simulink model "solarfuzzympptbldcmotorbattery"  (R2016a)
settings: Solver=ode45  StartTime=0.0  StopTime=1  RelTol=1e-3
undefined symbols (not defined in the file): Ion, Lithium
libraries: powerlib x32, simulink x13, electricdrivelib x1, fuzblock x1
settings Model: Creator=sudheer  LastModifiedBy=sudheer
settings SolverCC: ZeroCrossAlgorithm=Adaptive

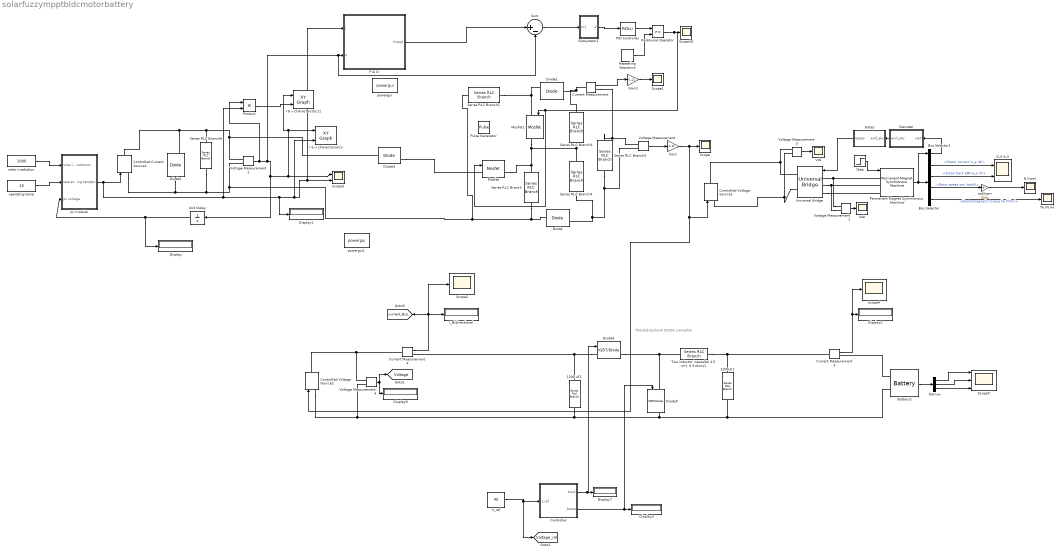
== system solarfuzzympptbldcmotorbattery ==
  note: The bidirectional DC/DC converter
  1200 uF1 : powerlib/Elements/Series RLC Branch  LConnTagsString=__new0  RConnTagsString=__new0  BranchType=RC  Resistance=0.001  Inductance=3e-3  SetiL0=off  InitialCurrent=0  Capacitance=1200e-6  Setx0=off  InitialVoltage=0  Measurements=None
  1200uF1 : powerlib/Elements/Series RLC Branch  LConnTagsString=__new0  RConnTagsString=__new0  BranchType=C  Resistance=1  Inductance=3e-3  SetiL0=off  InitialCurrent=0  Capacitance=1200e-6  Setx0=off  InitialVoltage=0  Measurements=None
  Battery2 : electricdrivelib/Extra Sources/Battery  BatType=Lithium-Ion  ShowTempParam=off  ThermalPreset=no  NomV=200  NomQ=100  SOC=80  Batt_Tr=0.1  PresetModel=on  MaxQ=100  MinV=150  FullV=232.7974  Dis_rate=43.4783  R=0.02  Normal_OP=90.4348  expZone="[216.0772      4.913043]"  current=[1.5 3]  Units=Ampere-hour  Tci=20  NomT=20  T2=-30  MaxQ2=4.8  FullV2=7.1  Normal_OP2=5.72  expZone2="[6.58  1]"  Rca=0.6  ti=1000  Dp=0
  Bus Selector : BusSelector  OutputSignals=Stator current is_a (A),Stator back EMF e_a (V),Rotor speed wm (rad/s),Electromagnetic torque Te (N*m)
  Bus Selector1 : BusSelector  OutputSignals=Hall effect signal h_a,Hall effect signal h_b,Hall effect signal h_c  OutputAsBus=on
  Controlled Current Source1 : powerlib/Electrical Sources/Controlled Current Source  Initialize=on  Source_Type=AC  Amplitude=0  Phase=0  Frequency=0  Measurements=None
  Controlled Voltage Source1 : powerlib/Electrical Sources/Controlled Voltage Source  Initialize=on  Source_Type=AC  Amplitude=500  Phase=0  Frequency=0  Measurements=None
  Controlled Voltage Source2 : powerlib/Electrical Sources/Controlled Voltage Source  Initialize=on  Source_Type=AC  Amplitude=500  Phase=0  Frequency=0  Measurements=None
  Controller : Subsystem
  Current Measurement : powerlib/Measurements/Current Measurement  PhasorSimulation=off  OutputType=Complex  PSBequivalent=0
  Current Measurement3 : powerlib/Measurements/Current Measurement  PhasorSimulation=off  OutputType=Complex  PSBequivalent=0
  Current Measurement4 : powerlib/Measurements/Current Measurement  PhasorSimulation=off  OutputType=Complex  PSBequivalent=0
  Decoder : Subsystem
  Demux : Demux  Outputs=3
  Diode{,1..3} (4 alike) : powerlib/Power Electronics/Diode  Ron=0.001  Lon=0  Vf=0.8  IC=0  UseSnubber=off  Rs=500  Cs=250e-9  Measurements=on
  Diode4 : powerlib/Power Electronics/IGBT//Diode  Ron=1e-3  Rs=1e5  Cs=inf  Measurements=on
  Diode5 : powerlib/Power Electronics/IGBT//Diode  Ron=1e-3  Rs=1e5  Cs=inf  Measurements=on
  Display{,1..3,7,9} (6 alike) : Display
  Gain : Gain  Gain=-1.11
  Gain1 : Gain  Gain=-1.11
  Gates : Subsystem
  I & v characteristics : simulink/Sinks/XY Graph  xmin=0  xmax=100  ymin=0  ymax=15  st=-1
  I & v characteristics1 : simulink/Sinks/XY Graph  xmin=0  xmax=100  ymin=0  ymax=1000  st=-1
  I_Bidirectional : Display
  Mosfet : powerlib/Power Electronics/Mosfet  Ron=0.1  Lon=0  Rd=0.01  Vfd=0  IC=0  Rs=1e5  Cs=inf  Measurements=on
  Mosfet1 : powerlib/Power Electronics/Mosfet  Ron=0.1  Lon=0  Rd=0.01  Vfd=0  IC=0  Rs=1e5  Cs=inf  Measurements=on
  N (rpm) : Scope
  P & O : Subsystem
  PID Controller : simulink/Continuous/PID Controller  Controller=PID  TimeDomain=Continuous-time  SampleTime=-1  IntegratorMethod=Forward Euler  FilterMethod=Forward Euler  Form=Parallel  UseFilter=on  ControllerParametersSource=internal  P=65  I=1300  D=1.1  N=1000  InitialConditionSource=internal  InitialConditionForIntegrator=0  InitialConditionForFilter=0  ExternalReset=none  LimitOutput=on  UpperSaturationLimit=0.9  LowerSaturationLimit=0.1  LinearizeAsGain=on  AntiWindupMode=none  Kb=1  TrackingMode=off  Kt=1  PParamMin=[]  PParamMax=[]  IParamMin=[]  IParamMax=[]  DParamMin=[]  DParamMax=[]  NParamMin=[]  NParamMax=[]  KbParamMin=[]  KbParamMax=[]  KtParamMin=[]  KtParamMax=[]  POutMin=[]  POutMax=[]  IOutMin=[]  IOutMax=[]  DOutMin=[]  DOutMax=[]  NOutMin=[]  NOutMax=[]  KbOutMin=[]  KbOutMax=[]  KtOutMin=[]  KtOutMax=[]  IntegratorOutMin=[]  IntegratorOutMax=[]  FilterOutMin=[]  FilterOutMax=[]  SumOutMin=[]  SumOutMax=[]  SumI1OutMin=[]  SumI1OutMax=[]  SumI2OutMin=[]  SumI2OutMax=[]  SumI3OutMin=[]  SumI3OutMax=[]  SumDOutMin=[]  SumDOutMax=[]  SaturationOutMin=[]  SaturationOutMax=[]  IntegratorContinuousStateAttributes=''  IntegratorStateMustResolveToSignalObject=off  IntegratorRTWStateStorageClass=Auto  FilterContinuousStateAttributes=''  FilterStateMustResolveToSignalObject=off  FilterRTWStateStorageClass=Auto  DifferentiatorICPrevScaledInput=0  DifferentiatorOutMin=[]  DifferentiatorOutMax=[]
  Permanent Magnet Synchronous Machine : powerlib/Machines/Permanent Magnet Synchronous Machine  NbPhases=3  FluxDistribution=Trapezoidal  RotorType=Round  MechanicalLoad=Torque Tm  PresetModel=No  ShowDetailedParameters=on  MeasurementBus=off  Resistance=2.8750  Inductance=8.5e-3  dqInductances=[8.5e-3, 8.5e-3]  La=0.000835  MachineConstant=Flux linkage established by magnets (V.s)  Flux=0.175  VoltageCst=146.6077  TorqueCst=1.4  Flat=120  Mechanical=[ 0.8e-3, 1e-3 4]  PolePairs=4  InitialConditions=[0,0, 0,0]  InitialConditions5ph=[0 0 0 0 0 0]  TsPowergui=0  TsBlock=-1  RefAngle=90 degrees behind phase A axis (modified Park)
  Product : Product
  Pulse Generator : DiscretePulseGenerator  PulseType=Time based  Period=1/24000  PulseWidth=70
  Relational Operator : RelationalOperator  OutDataTypeStr=boolean
  Repeating Sequence : simulink/Sources/Repeating Sequence  rep_seq_t=[0 1 2 3 4 ]*(1/3e3)  rep_seq_y=[0 1 0 -1 0]
  Scope{,1..2,4,16} (5 alike) : Scope
  Scope3 : Scope  NumInputPorts=2
  Scope5 : Scope  NumInputPorts=3
  Series RLC Branch : powerlib/Elements/Series RLC Branch  LConnTagsString=__new0  RConnTagsString=__new0  BranchType=L  Resistance=1  Inductance=1e-3  SetiL0=off  InitialCurrent=0  Capacitance=1e-6  Setx0=off  InitialVoltage=0  Measurements=None
  Series RLC Branch1 : powerlib/Elements/Series RLC Branch  LConnTagsString=__new0  RConnTagsString=__new0  BranchType=C  Resistance=1  Inductance=1e-3  SetiL0=off  InitialCurrent=0  Capacitance=500e-6  Setx0=off  InitialVoltage=0  Measurements=None
  Series RLC Branch2 : powerlib/Elements/Series RLC Branch  LConnTagsString=__new0  RConnTagsString=__new0  BranchType=R  Resistance=100  Inductance=1e-3  SetiL0=off  InitialCurrent=0  Capacitance=1e-6  Setx0=off  InitialVoltage=0  Measurements=None
  Series RLC Branch3 : powerlib/Elements/Series RLC Branch  LConnTagsString=__new0  RConnTagsString=__new0  BranchType=C  Resistance=1  Inductance=1e-3  SetiL0=off  InitialCurrent=0  Capacitance=300e-6  Setx0=off  InitialVoltage=0  Measurements=None
  Series RLC Branch4 : powerlib/Elements/Series RLC Branch  LConnTagsString=__new0  RConnTagsString=__new0  BranchType=C  Resistance=1  Inductance=1e-3  SetiL0=off  InitialCurrent=0  Capacitance=300e-6  Setx0=off  InitialVoltage=0  Measurements=None
  Series RLC Branch6 : powerlib/Elements/Series RLC Branch  LConnTagsString=__new0  RConnTagsString=__new0  BranchType=C  Resistance=1  Inductance=1e-3  SetiL0=off  InitialCurrent=0  Capacitance=1000e-6  Setx0=on  InitialVoltage=0  Measurements=None
  Step : Step  Time=.1  After=3  SampleTime=0
  Subsystem1 : Subsystem
  Sum : Sum  Inputs=|+-
  Te (N.m) : Scope
  "Two inductor inparallel 4.5 mH, 0.3 ohms1" : powerlib/Elements/Series RLC Branch  LConnTagsString=__new0  RConnTagsString=__new0  BranchType=RL  Resistance=.25  Inductance=4.5e-3  SetiL0=off  InitialCurrent=0  Capacitance=1e-6  Setx0=off  InitialVoltage=0  Measurements=None
  Unit Delay : UnitDelay  SampleTime=-1
  Universal Bridge : powerlib/Power Electronics/Universal Bridge  Arms=3  SnubberResistance=5000  SnubberCapacitance=1e-6  Device=MOSFET / Diodes  Ron=1e-3  Lon=0  ForwardVoltages="[  0  0  ]"  ForwardVoltage=0  GTOparameters=[ 10e-6 , 20e-6 ]  IGBTparameters=[ 1e-6 , 2e-6 ]  Measurements=None  Measurements_2=None  converterType=Rectifier
  V_ref : Constant  Value=45
  Vab : Scope
  Vdc : Scope
  Voltage Measurement{,1..4} (5 alike) : powerlib/Measurements/Voltage Measurement  PhasorSimulation=off  OutputType=Complex  PSBequivalent=0
  is_a e_a : Scope  NumInputPorts=2
  operating temp : Constant  Value=25
  powergui : powerlib/powergui  Priority=1  SimulationMode=Discrete  SolverType=Tustin/Backward Euler (TBE)  SampleTime=50e-6  frequency=60  SPID=off  DisableSnubberDevices=off  DisableRonSwitches=off  DisableVfSwitches=off  SwTol=0  DisplayEquations=off  Interpol=off  ExternalGateDelay=off  methode=off  Ts=10  FunctionMessages=off  echomessages=off  HookPort=off  EnableUseOfTLC=off  x0status=blocks  frequencyindice=0  Pbase=100e6  ErrMax=1e-4  Iterations=50  UnitsV=kV  UnitsW=MW  buscounter=0  RestoreLinks=warning  ResistiveCurrentMeasurement=off  Frange=[0:2:500]  Ylog=off  Xlog=on  ShowGrid=off  save=off  variable=ZData  structure=0  ZoomFFT=off  StartTime=0.0  cycles=1  DisplayStyle=1  fundamental=60  FreqAxis=off  MaxFrequency=1000  frequencyindicesteady=1  RmsSteady=1  display=off
  powergui1 : powerlib/powergui  Priority=1  SimulationMode=Discrete  SolverType=Backward Euler  SampleTime=1e-5  frequency=60  SPID=off  DisableSnubberDevices=off  DisableRonSwitches=off  DisableVfSwitches=off  SwTol=0  DisplayEquations=off  Interpol=off  ExternalGateDelay=off  methode=off  Ts=0  FunctionMessages=off  echomessages=off  HookPort=off  EnableUseOfTLC=off  x0status=blocks  frequencyindice=0  Pbase=100e6  ErrMax=1e-4  Iterations=50  UnitsV=kV  UnitsW=MW  buscounter=0  RestoreLinks=warning  ResistiveCurrentMeasurement=off  Frange=[0:2:500]  Ylog=off  Xlog=on  ShowGrid=off  save=off  variable=ZData  structure=0  ZoomFFT=off  StartTime=0.0  cycles=1  DisplayStyle=1  fundamental=60  FreqAxis=off  MaxFrequency=1000  frequencyindicesteady=1  RmsSteady=1  display=off
  pv module : Subsystem  mask{Voc=60, Isc=9.4, Ns=100, Np=1, Rsh=1000, Rs=0.0001}
      mask prompts: Voc "open circuit voltage"; Isc "shortcircuit current"; Ns "modules in series"; Np "modules in parallel"; Rsh "shunt resistance"; Rs "series resistance"
  rad2rpm : Gain  Gain=30/pi
  solar irradiation : Constant  Value=1000
  tag scope: Voltage=global, Voltage_ref=global, current_Bus=global
  wires:
  Voltage Measurement/1 -> Gain/1
  Current Measurement/1 -> Gain1/1
  Gain/1 -> Controlled Voltage Source2/1, Controlled Voltage Source1/1, Scope/1
  solar irradiation/1 -> pv module/1(solar irradiation)
  operating temp/1 -> pv module/2(operating temp)
  Voltage Measurement1/1 -> Product/1, Sum/2, P & O/2(V), I & v characteristics/1, I & v characteristics1/1, Scope3/1, Unit Delay/1
  Unit Delay/1 -> Display/1, pv module/3(pv voltage)
  pv module/1(Ipv) -> Display1/1, I & v characteristics/2, Scope3/2, P & O/1(I), Product/2, Controlled Current Source1/1
  P & O/1(Vmpp1) -> Sum/1
  Relational Operator/1 -> Mosfet/1, Mosfet1/1, Scope16/1
  Sum/1 -> Subsystem1/1(In1)
  Repeating Sequence/1 -> Relational Operator/2
  PID Controller/1 -> Relational Operator/1
  Subsystem1/1(Out1) -> PID Controller/1
  Step/1 -> Permanent Magnet Synchronous Machine/1
  Gates/1(Gates) -> Universal Bridge/1
  Decoder/1(emf_abc) -> Gates/1("emf_abc ")
  rad2rpm/1 -> N (rpm)/1
  Voltage Measurement2/1 -> Vab/1
  Voltage Measurement3/1 -> Vdc/1
  Bus Selector/1 -> is_a e_a/1  "<Stator current is_a (A)>"
  Permanent Magnet Synchronous Machine/1 -> Bus Selector/1, Bus Selector1/1
  Bus Selector1/1 -> Decoder/1("Hall ")
  Bus Selector/2 -> is_a e_a/2  "<Stator back EMF e_a (V)>"
  Bus Selector/3 -> rad2rpm/1  "<Rotor speed wm (rad/s)>"
  Bus Selector/4 -> Te (N.m)/1  "<Electromagnetic torque Te (N*m)>"
  Current Measurement3/1 -> Display2/1, Scope4/1
  Controller/2(boost) -> Diode5/1, Display3/1
  Controller/1(buck) -> Diode4/1, Display7/1
  Current Measurement4/1 -> [current_Bus], Scope2/1, I_Bidirectional/1
  Voltage Measurement4/1 -> Display9/1, [Voltage]
  V_ref/1 -> [Voltage_ref], Controller/1(I_ref)
  Battery2/1 -> Demux/1
  Demux/1 -> Scope5/1
  Demux/2 -> Scope5/2
  Demux/3 -> Scope5/3
  Gain1/1 -> Scope1/1
  Product/1 -> I & v characteristics1/2
  connections:
  Voltage Measurement4/LConn1 -- Current Measurement4/LConn1 -- Controlled Voltage Source2/RConn1
  Series RLC Branch1/RConn1 -- Diode1/RConn1 -- Mosfet1/LConn1
  Universal Bridge/RConn1 -- Controlled Voltage Source1/RConn1 -- Voltage Measurement3/LConn1
  Series RLC Branch2/RConn1 -- Voltage Measurement/LConn2 -- Series RLC Branch4/LConn1 -- Diode/RConn1
  Current Measurement/LConn1 -- Series RLC Branch3/RConn1 -- Diode1/LConn1
  Diode5/RConn1 -- Controlled Voltage Source2/LConn1 -- Voltage Measurement4/LConn2 -- 1200 uF1/RConn1 -- Battery2/LConn2 -- 1200uF1/RConn1
  Controlled Current Source1/RConn1 -- Diode2/RConn1 -- Diode3/LConn1 -- Voltage Measurement1/LConn1 -- Series RLC Branch6/LConn1
  Diode3/RConn1 -- Mosfet/LConn1
  Voltage Measurement2/LConn1 -- Permanent Magnet Synchronous Machine/LConn1 -- Universal Bridge/LConn1
  Voltage Measurement2/LConn2 -- Permanent Magnet Synchronous Machine/LConn2 -- Universal Bridge/LConn2
  Universal Bridge/LConn3 -- Permanent Magnet Synchronous Machine/LConn3
  Series RLC Branch2/LConn1 -- Current Measurement/RConn1 -- Voltage Measurement/LConn1
  Universal Bridge/RConn2 -- Controlled Voltage Source1/LConn1 -- Voltage Measurement3/LConn2
  "Two inductor inparallel 4.5 mH, 0.3 ohms1"/LConn1 -- Diode5/LConn1 -- Diode4/RConn1
  1200uF1/LConn1 -- Current Measurement3/LConn1 -- "Two inductor inparallel 4.5 mH, 0.3 ohms1"/RConn1
  Diode4/LConn1 -- 1200 uF1/LConn1 -- Current Measurement4/RConn1
  Battery2/LConn1 -- Current Measurement3/RConn1
  Mosfet/RConn1 -- Mosfet1/RConn1 -- Series RLC Branch3/LConn1 -- Series RLC Branch4/RConn1 -- Series RLC Branch/LConn1
  Voltage Measurement1/LConn2 -- Series RLC Branch/RConn1 -- Diode/LConn1 -- Series RLC Branch1/LConn1 -- Series RLC Branch6/RConn1 -- Diode2/LConn1 -- Controlled Current Source1/LConn1

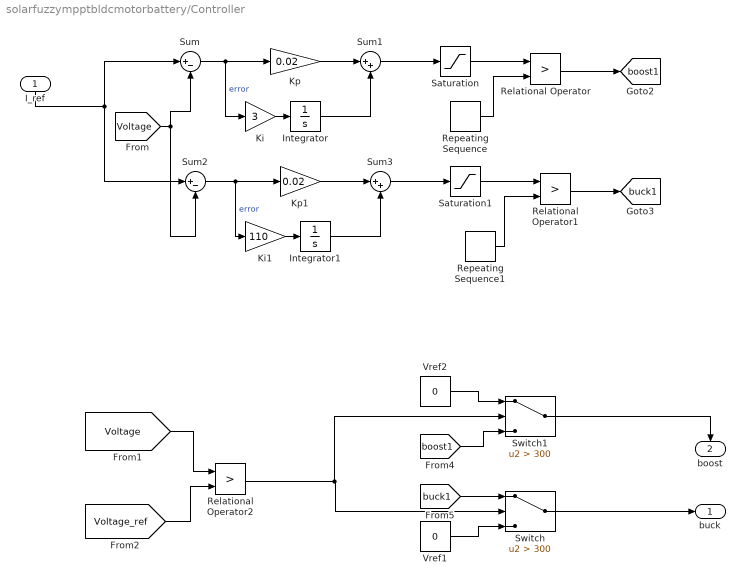
== system solarfuzzympptbldcmotorbattery/Controller ==
  I_ref : Inport
  Integrator : Integrator  LimitOutput=on  UpperSaturationLimit=0.9  LowerSaturationLimit=0
  Integrator1 : Integrator  LimitOutput=on  UpperSaturationLimit=0.9  LowerSaturationLimit=0
  Ki : Gain  Gain=3
  Ki1 : Gain  Gain=110
  Kp : Gain  Gain=0.02
  Kp1 : Gain  Gain=0.02
  Relational Operator : RelationalOperator  Operator=>  OutDataTypeStr=boolean
  Relational Operator1 : RelationalOperator  Operator=>  OutDataTypeStr=boolean
  Relational Operator2 : RelationalOperator  Operator=>  OutDataTypeStr=boolean
  Repeating Sequence : simulink/Sources/Repeating Sequence  rep_seq_t=[0 1/5000]  rep_seq_y=[0 1]
  Repeating Sequence1 : simulink/Sources/Repeating Sequence  rep_seq_t=[0 1/5000]  rep_seq_y=[0 1]
  Saturation : Saturate  UpperLimit=0.9  LowerLimit=0
  Saturation1 : Saturate  UpperLimit=0.9  LowerLimit=0
  Sum : Sum  Inputs=|+-
  Sum1 : Sum  Inputs=|++
  Sum2 : Sum  Inputs=|+-
  Sum3 : Sum  Inputs=|++
  Switch : Switch  Criteria=u2 > Threshold  Threshold=300
  Switch1 : Switch  Criteria=u2 > Threshold  Threshold=300
  Vref1 : Constant  Value=0
  Vref2 : Constant  Value=0
  buck : Outport
  boost : Outport  Port=2
  tag scope: boost1=global, buck1=global
  wires:
  Switch/1 -> buck/1
  [boost1] -> Switch1/3
  Switch1/1 -> boost/1
  Ki1/1 -> Integrator1/1
  Saturation1/1 -> Relational Operator1/1
  Saturation/1 -> Relational Operator/1
  Sum2/1 -> Kp1/1, Ki1/1  "error"
  Relational Operator1/1 -> [buck1]
  Kp1/1 -> Sum3/1
  [Voltage] -> Sum2/2, Sum/2
  Repeating Sequence1/1 -> Relational Operator1/2
  Repeating Sequence/1 -> Relational Operator/2
  Integrator1/1 -> Sum3/2
  Sum3/1 -> Saturation1/1
  Ki/1 -> Integrator/1
  Sum1/1 -> Saturation/1
  I_ref/1 -> Sum/1, Sum2/1
  Relational Operator/1 -> [boost1]
  Sum/1 -> Ki/1, Kp/1  "error"
  Kp/1 -> Sum1/1
  Integrator/1 -> Sum1/2
  Vref2/1 -> Switch1/1
  Vref1/1 -> Switch/3
  [buck1] -> Switch/1
  [Voltage] -> Relational Operator2/1
  [Voltage_ref] -> Relational Operator2/2
  Relational Operator2/1 -> Switch1/2, Switch/2

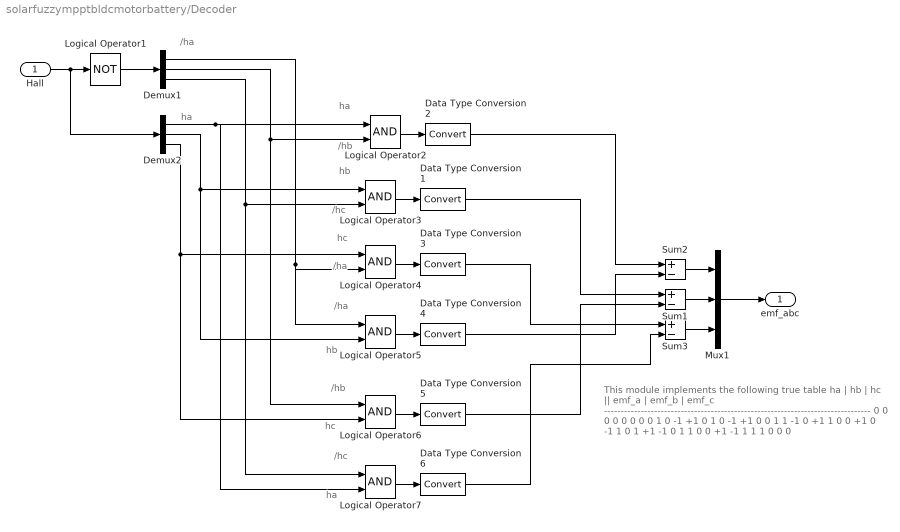
== system solarfuzzympptbldcmotorbattery/Decoder ==
  note: /ha
  note: ha
  note: ha
  note: /hb
  note: hb
  note: /hc
  note: hc
  note: /ha
  note: /ha
  note: hb
  note: /hb
  note: hc
  note: /hc
  note: ha
  note: This module implements the following true table
      |
      |    ha   |   hb   |   hc   ||   emf_a   |   emf_b   |   emf_c
      |     --------------------------------------------------------------------------------
      | 0          0         0          0               0               0
      | 0          0         1          0               -1              +1
      | 0          1         0          -1              +1                0
      | 0          1         1          -1               0               +1
      | 1          0         0         +1               0               -1
      | 1          0         1         +1              -1                0
      | 1          1         0          0              +1               -1
      | 1          1         1          0               0                0
  "Hall " : Inport
  Data Type Conversion{1..6} (6 alike) : DataTypeConversion
  Demux1 : Demux  Outputs=3
  Demux2 : Demux  Outputs=3
  Logical Operator1 : Logic  Operator=NOT  AllPortsSameDT=off  OutDataTypeStr=boolean
  Logical Operator{2..7} (6 alike) : Logic  AllPortsSameDT=off  OutDataTypeStr=boolean
  Mux1 : Mux  Inputs=3
  Sum1 : Sum  Inputs=+-  OutDataTypeStr=double
  Sum2 : Sum  Inputs=+-  OutDataTypeStr=double
  Sum3 : Sum  Inputs=+-  OutDataTypeStr=double
  emf_abc : Outport
  wires:
  "Hall "/1 -> Logical Operator1/1, Demux2/1
  Logical Operator1/1 -> Demux1/1
  Demux2/3 -> Logical Operator4/1, Logical Operator6/2
  Demux2/2 -> Logical Operator3/1, Logical Operator5/2
  Demux2/1 -> Logical Operator2/1, Logical Operator7/2
  Demux1/3 -> Logical Operator3/2, Logical Operator7/1
  Demux1/2 -> Logical Operator2/2, Logical Operator6/1
  Demux1/1 -> Logical Operator4/2, Logical Operator5/1
  Logical Operator2/1 -> Data Type Conversion2/1
  Sum2/1 -> Mux1/1
  Sum1/1 -> Mux1/2
  Sum3/1 -> Mux1/3
  Mux1/1 -> emf_abc/1
  Logical Operator3/1 -> Data Type Conversion1/1
  Logical Operator4/1 -> Data Type Conversion3/1
  Logical Operator5/1 -> Data Type Conversion4/1
  Logical Operator6/1 -> Data Type Conversion5/1
  Logical Operator7/1 -> Data Type Conversion6/1
  Data Type Conversion2/1 -> Sum2/1
  Data Type Conversion4/1 -> Sum2/2
  Data Type Conversion1/1 -> Sum1/1
  Data Type Conversion5/1 -> Sum1/2
  Data Type Conversion3/1 -> Sum3/1
  Data Type Conversion6/1 -> Sum3/2

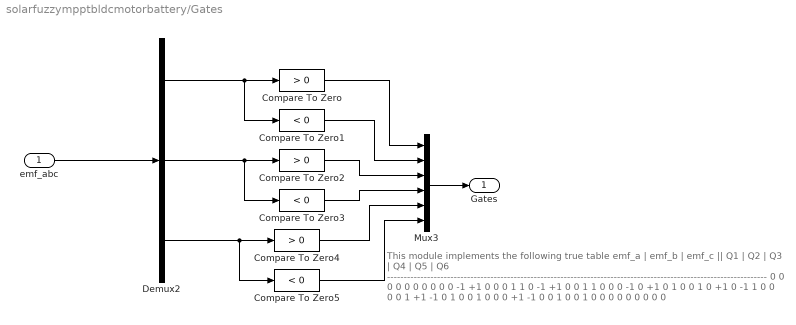
== system solarfuzzympptbldcmotorbattery/Gates ==
  note: This module implements the following true table
      |
      |    emf_a   |   emf_b   |   emf_c   ||   Q1   |   Q2   |   Q3   |   Q4   |   Q5   |   Q6
      |     ------------------------------------------------------------------------------------------------------------------
      |       0              0                0            0          0          0           0        0        0
      |       0               -1              +1          0          0          0           1        1        0
      |     -1              +1                0          0          1          1           0        0        0
      |     -1               0               +1          0          1         0           0        1        0
      |    +1               0                -1          1          0          0           0        0        1
      |    +1              -1                0           1          0          0           1        0        0
      |      0              +1               -1           0          0          1           0        0        1
      |     0              0                0             0          0          0           0        0        0
  "emf_abc " : Inport
  Compare To Zero : simulink/Logic and Bit Operations/Compare To Zero  relop=>  OutDataTypeStr=boolean  ZeroCross=off
  Compare To Zero1 : simulink/Logic and Bit Operations/Compare To Zero  relop=<  OutDataTypeStr=boolean  ZeroCross=off
  Compare To Zero2 : simulink/Logic and Bit Operations/Compare To Zero  relop=>  OutDataTypeStr=boolean  ZeroCross=off
  Compare To Zero3 : simulink/Logic and Bit Operations/Compare To Zero  relop=<  OutDataTypeStr=boolean  ZeroCross=off
  Compare To Zero4 : simulink/Logic and Bit Operations/Compare To Zero  relop=>  OutDataTypeStr=boolean  ZeroCross=off
  Compare To Zero5 : simulink/Logic and Bit Operations/Compare To Zero  relop=<  OutDataTypeStr=boolean  ZeroCross=off
  Demux2 : Demux  Outputs=3
  Mux3 : Mux  Inputs=6
  Gates : Outport
  wires:
  "emf_abc "/1 -> Demux2/1
  Mux3/1 -> Gates/1
  Demux2/1 -> Compare To Zero/1, Compare To Zero1/1
  Demux2/2 -> Compare To Zero2/1, Compare To Zero3/1
  Demux2/3 -> Compare To Zero4/1, Compare To Zero5/1
  Compare To Zero/1 -> Mux3/1
  Compare To Zero1/1 -> Mux3/2
  Compare To Zero2/1 -> Mux3/3
  Compare To Zero3/1 -> Mux3/4
  Compare To Zero4/1 -> Mux3/5
  Compare To Zero5/1 -> Mux3/6

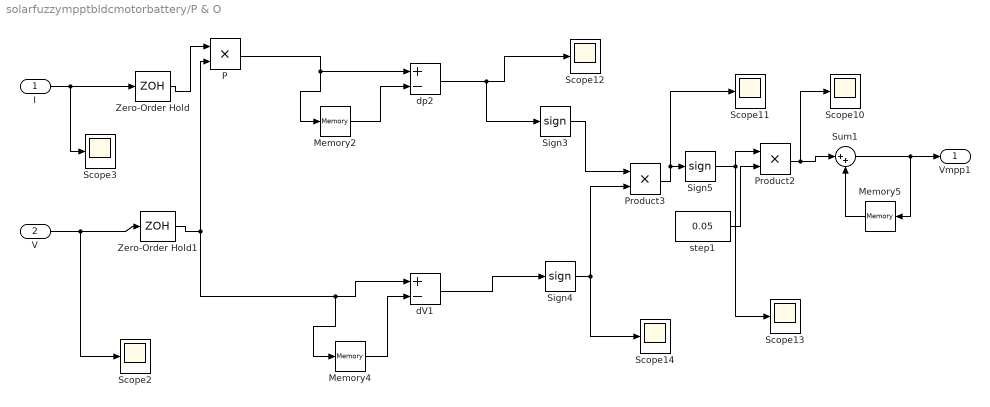
== system solarfuzzympptbldcmotorbattery/P & O ==
  I : Inport
  V : Inport  Port=2
  Memory2 : Memory  InheritSampleTime=on
  Memory4 : Memory  InheritSampleTime=on
  Memory5 : Memory  InheritSampleTime=on
  P : Product  RndMeth=Zero
  Product2 : Product  RndMeth=Zero
  Product3 : Product  RndMeth=Zero
  Scope{2..3,10..14} (7 alike) : Scope
  Sign3 : Signum
  Sign4 : Signum
  Sign5 : Signum
  Sum1 : Sum  Inputs=|++
  Zero-Order Hold : ZeroOrderHold  SampleTime=0.002
  Zero-Order Hold1 : ZeroOrderHold  SampleTime=0.002
  dV1 : Sum  Inputs=+-
  dp2 : Sum  Inputs=+-
  step1 : Constant  Value=0.05
  Vmpp1 : Outport
  wires:
  V/1 -> Zero-Order Hold1/1, Scope2/1
  I/1 -> Zero-Order Hold/1, Scope3/1
  Zero-Order Hold/1 -> P/1
  P/1 -> Memory2/1, dp2/1
  Memory2/1 -> dp2/2
  Zero-Order Hold1/1 -> P/2, Memory4/1, dV1/1
  Memory4/1 -> dV1/2
  dV1/1 -> Sign4/1
  step1/1 -> Product2/2
  Product2/1 -> Sum1/1, Scope10/1
  Sign3/1 -> Product3/1
  Sign4/1 -> Product3/2, Scope14/1
  Product3/1 -> Sign5/1, Scope11/1
  dp2/1 -> Sign3/1, Scope12/1
  Sign5/1 -> Product2/1, Scope13/1
  Sum1/1 -> Memory5/1, Vmpp1/1
  Memory5/1 -> Sum1/2

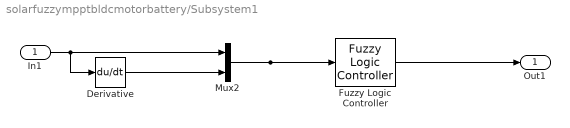
== system solarfuzzympptbldcmotorbattery/Subsystem1 ==
  In1 : Inport
  Derivative : Derivative
  Fuzzy Logic Controller : fuzblock/Fuzzy Logic  Controller  fis=saf
  Mux2 : Mux  Inputs=2
  Out1 : Outport
  wires:
  In1/1 -> Derivative/1, Mux2/1
  Derivative/1 -> Mux2/2
  Fuzzy Logic Controller/1 -> Out1/1
  Mux2/1 -> Fuzzy Logic Controller/1

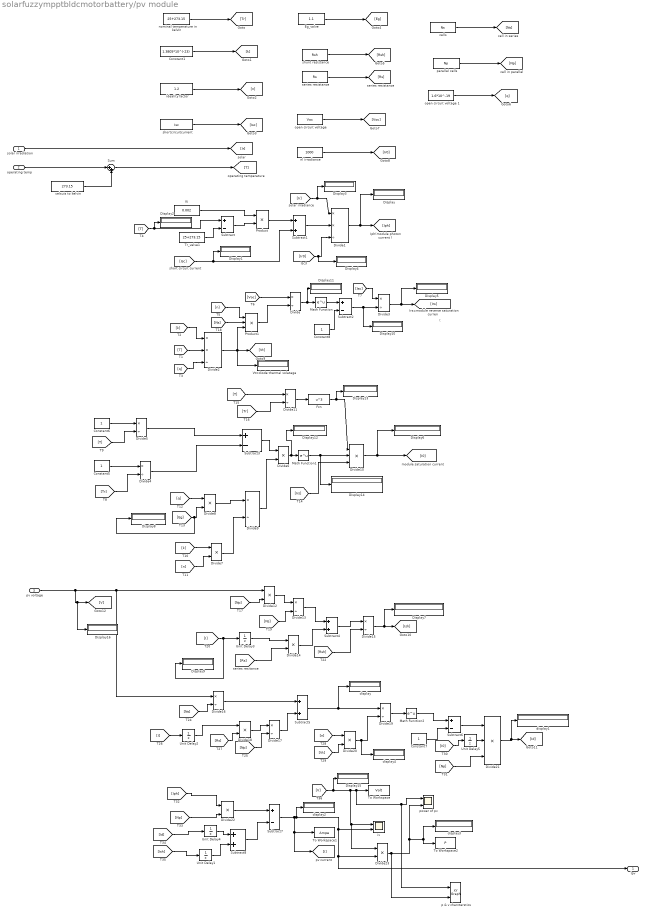
== system solarfuzzympptbldcmotorbattery/pv module ==
  note: t
  solar irradiation : Inport
  operating temp : Inport  Port=2
  pv voltage : Inport  Port=3
  Constant1 : Constant  Value=1.3805*10^(-23)
  Constant{5..8} (4 alike) : Constant
  Display{,1..16} (17 alike) : Display
  Divide{,3..5,9,11,13,15..17,19} (11 alike) : Product  Inputs=*/
  Divide1 : Product  Inputs=**/
  Divide10 : Product  Inputs=***
  Divide{6..8,12,14,18,20,22..23} (9 alike) : Product  Inputs=**
  Divide2 : Product  Inputs=**/
  Divide21 : Product  Inputs=***
  "Eg_valve " : Constant  Value=1.1
  Fcn : Fcn  Expr=u^3
  Ki : Constant  Value=0.002
  Math Function : Math  SaturateOnIntegerOverflow=on
  Math Function1 : Math  SaturateOnIntegerOverflow=on
  Math Function2 : Math  SaturateOnIntegerOverflow=on
  Product : Product
  Product1 : Product  Inputs=3
  Subtract{,2..3,6..7} (5 alike) : Sum  Inputs=+-
  Subtract{1,4..5,8} (4 alike) : Sum
  Sum : Sum  Inputs=|++
  To Workspace : ToWorkspace  VariableName=Volt  SaveFormat=Timeseries  SampleTime=-1
  To Workspace1 : ToWorkspace  VariableName=Ampe  SaveFormat=Timeseries  SampleTime=-1
  To Workspace2 : ToWorkspace  VariableName=P  SaveFormat=Timeseries  SampleTime=-1
  Tr_valve1 : Constant  Value=25+273.15
  Unit Delay{1..5} (5 alike) : UnitDelay  SampleTime=-1
  Vt=diode thermal volatage : Display
  cells : Constant  Value=Ns
  celsuis to kelvin : Constant  Value=273.15
  display{,1..4} (5 alike) : Display
  ideality factor : Constant  Value=1.2
  iv : Scope  NumInputPorts=2
  nl irradiance : Constant  Value=1000
  "nominal temperature in kelvin " : Constant  Value=25+273.15
  "open circuit voltage " : Constant  Value=Voc
  open circuit voltage 1 : Constant  Value=1.6*10^-19
  "p & v charcterstics " : simulink/Sinks/XY Graph  xmin=0  xmax=30  ymin=0  ymax=200  st=-1
  parallel cells : Constant  Value=Np
  power of pv : Scope  NumInputPorts=2
  series resistance : Constant  Value=Rs
  "shortcircuitcurrent " : Constant  Value=Isc
  "shunt resistance " : Constant  Value=Rsh
  Ipv : Outport
  wires:
  Subtract7/1 -> display2/1, Ipv/1, Divide23/2, iv/2, To Workspace1/1, [I]
  Divide10/1 -> Display6/1, [I0]
  Math Function/1 -> Subtract2/1
  Divide6/1 -> Display12/1, Math Function1/1
  [n] -> Product1/1
  [n] -> Divide7/2
  Constant8/1 -> Subtract2/2
  Constant5/1 -> Divide4/1
  [T] -> Divide11/1
  Subtract5/1 -> display/1, Divide19/1
  [Np] -> Divide17/2
  Divide11/1 -> Fcn/1
  [V] -> Display15/1, Divide23/1, iv/1, "p & v charcterstics "/1, power of pv/1, To Workspace/1
  Product/1 -> Subtract1/1
  Math Function1/1 -> Display14/1, Divide10/2
  Constant7/1 -> Subtract6/2
  [k] -> Divide2/1
  [Tr] -> Divide11/2
  "Eg_valve "/1 -> [Eg]
  Divide17/1 -> Subtract5/2
  [q] -> Divide2/3
  ideality factor/1 -> [n]
  Divide12/1 -> Divide13/1
  "shortcircuitcurrent "/1 -> [Isc]
  [Eg] -> Display8/1, Divide8/2
  [Isc] -> Divide3/1
  Ki/1 -> Product/1
  Subtract/1 -> Product/2
  [Tr] -> Divide4/2
  [q] -> Divide8/1
  Product1/1 -> Divide/2
  Subtract6/1 -> Divide21/1
  Constant1/1 -> [k]
  [n] -> Divide20/1
  solar irradiation/1 -> [Ir]
  Divide14/1 -> Subtract4/2
  Math Function2/1 -> Subtract6/1
  [Vt] -> Divide20/2
  Divide1/1 -> Display/1, [Iph]
  Subtract8/1 -> Subtract7/2
  Divide16/1 -> Subtract5/1
  [T] -> Divide2/2
  Divide15/1 -> Display7/1, [Ish]
  Divide18/1 -> Divide17/1
  [Rs] -> Divide18/2
  Subtract2/1 -> Display10/1, Divide3/2
  [Rsh] -> Divide15/2
  Fcn/1 -> Display13/1, Divide10/1
  Divide3/1 -> Display5/1, [Irs]
  pv voltage/1 -> Divide16/1, Divide12/1, Display16/1, [V]
  [Ir0] -> Display4/1, Divide1/3
  [Ns] -> Divide13/2
  Divide13/1 -> Subtract4/1
  [Np] -> Divide21/3
  Divide/1 -> Display11/1, Math Function/1
  [T] -> Display2/1, Subtract/1
  [Irs] -> Divide10/3
  [Np] -> Divide22/2
  Divide21/1 -> display1/1, [Id]
  Divide2/1 -> Product1/3, Vt=diode thermal volatage/1, [Vt]
  Divide22/1 -> Subtract7/1
  [Voc] -> Divide/1
  "shunt resistance "/1 -> [Rsh]
  Divide9/1 -> Divide6/2
  Tr_valve1/1 -> Subtract/2
  [k] -> Divide7/1
  Divide20/1 -> display4/1, Divide19/2
  Divide19/1 -> Math Function2/1
  "open circuit voltage "/1 -> [Voc]
  Subtract4/1 -> Divide15/1
  [Np] -> Divide12/2
  [Ns] -> Divide16/2
  [Rs] -> Divide14/2
  Subtract3/1 -> Divide6/1
  [Isc] -> Display1/1, Subtract1/2
  Subtract1/1 -> Divide1/2
  [Ir] -> Display3/1, Divide1/1
  "nominal temperature in kelvin "/1 -> [Tr]
  [Iph] -> Divide22/1
  [Ish] -> Unit Delay1/1
  Unit Delay1/1 -> Subtract8/2
  [I] -> Unit Delay2/1
  Unit Delay2/1 -> Divide18/1
  open circuit voltage 1/1 -> [q]
  cells/1 -> [Ns]
  parallel cells/1 -> [Np]
  series resistance/1 -> [Rs]
  nl irradiance/1 -> [Ir0]
  [I] -> Display9/1, Unit Delay3/1
  [Ns] -> Product1/2
  Constant6/1 -> Divide5/1
  [T] -> Divide5/2
  Divide8/1 -> Divide9/1
  Divide7/1 -> Divide9/2
  Divide5/1 -> Subtract3/1
  Divide4/1 -> Subtract3/2
  Unit Delay3/1 -> Divide14/1
  [Id] -> Unit Delay4/1
  Unit Delay4/1 -> Subtract8/1
  Unit Delay5/1 -> Divide21/2
  [I0] -> Unit Delay5/1
  operating temp/1 -> Sum/1
  Sum/1 -> [T]
  celsuis to kelvin/1 -> Sum/2
  Divide23/1 -> "p & v charcterstics "/2, display3/1, To Workspace2/1, power of pv/2
